simulink library "user_lib"  (R2022b)
settings: Solver=VariableStepAuto  StartTime=0.0  StopTime=10.0  RelTol=1e-3
libraries: simulink x5
settings Model: Creator=MBDUSR  LastModifiedBy=MBDUSR

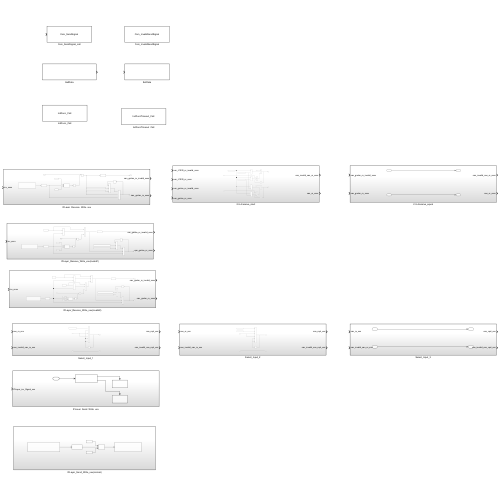
[thumbnail: Simulink's stored preview of the top-level diagram]
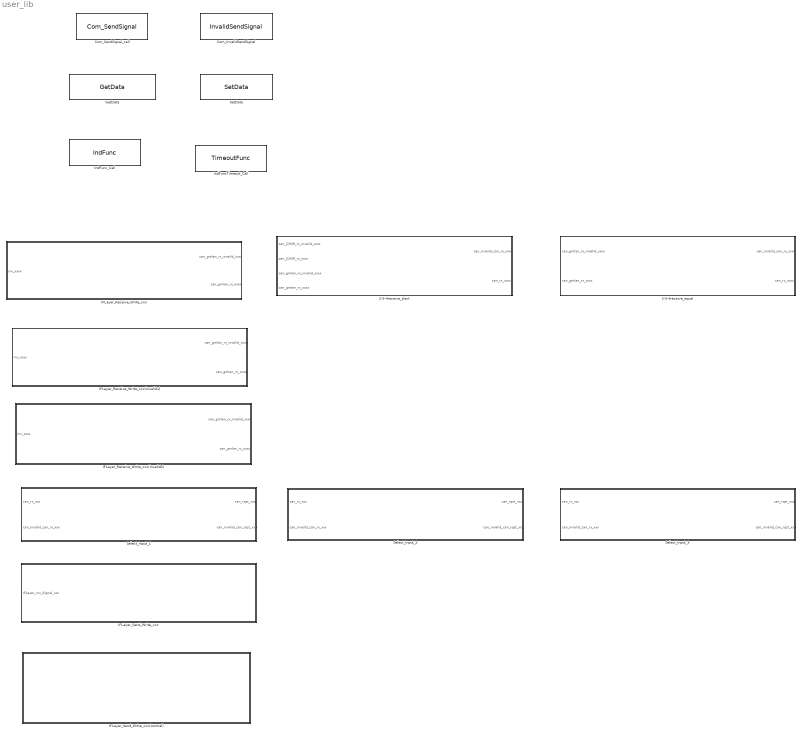
== system user_lib ==
  2-5-4receive_equal : Subsystem
  2-5-4receive_slect : Subsystem
  Com_InvalidSendSignal : S-Function  FunctionName=InvalidSendSignal  Parameters=signalId  SFunctionDeploymentMode=off  EnableBusSupport=off  mask{signalId=}
      mask Help: web('Com_InvalidSendSignal_help.html')
      mask DialogControl Container4 Prompt: Singal Parameter
      mask Display: disp('Com_InvalidSendSignal')
  Com_SendSignal_call : S-Function  FunctionName=Com_SendSignal  Parameters=signalId  SFunctionDeploymentMode=off  EnableBusSupport=off  mask{signalId=}
      mask Help: web('Com_SendSignal_help.html')
      mask DialogControl Container4 Prompt: Singal Parameter
      mask Display: disp('Com_SendSignal')
  GetData : S-Function  FunctionName=GetData  Parameters=interface,signalType  SFunctionDeploymentMode=off  EnableBusSupport=off  mask{interface=, signalType=UB}
      mask prompts: signalType "Signal Type"
      mask Help: web('GetData_help.html')
      mask TypeOptions signalType: UB | SB | UW | SW | UD | SD
      mask DialogControl Container4 Prompt: Singal Parameter
      mask Display:
      | interfaceName = get_param(gcbh, "interface");
      | s = strcat(interfaceName);
      | disp(s);
  IFLayer_Receive_Write_xxx : Subsystem
  IFLayer_Receive_Write_xxx(invalid1) : Subsystem
  IFLayer_Receive_Write_xxx(invalid2) : Subsystem
  IFLayer_Send_Write_xxx : Subsystem
  IFLayer_Send_Write_xxx(normal) : Subsystem
  IndFuncTimeout_Call : S-Function  FunctionName=TimeoutFunc  Parameters=siggroupIndex,canid,signalTable  SFunctionDeploymentMode=off  EnableBusSupport=off  mask{siggroupIndex=, canid=, signalTable={ 'UB', '', ''; 'UW', '', '' }}
      mask prompts: siggroupIndex "Signal Group Index"; canid "CAN ID"; signalTable "Signal Table"
      mask init:
      | %set_param(gcbh,'signalTable',{'1','signal1','index1'});
      mask Help: web('IndFuncTimeout_help.html')
      mask DialogControl Container4 Prompt: Singal Parameter
      mask Display: disp('IndFuncTimeout_Call')
  IndFunc_Call : S-Function  FunctionName=IndFunc  Parameters=siggroupIndex,canid,signalTable,timeoutflag,extendid  SFunctionDeploymentMode=off  EnableBusSupport=off  mask{siggroupIndex=, canid=, signalTable={ 'UB', '', ''; 'UB', '', '' }, timeoutflag=off, extendid=off}
      mask prompts: siggroupIndex "Signal Group Index"; canid "CAN ID"; signalTable "Signal Table"; timeoutflag "Timeout Flag"; extendid "Extend ID"
      mask init:
      | %set_param(gcbh,'signalTable',{'1','signal1','index1'});
      mask Help: web('IndFunc_help.html')
      mask DialogControl Container4 Prompt: Singal Parameter
      mask Display: disp('IndFunc_Call')
  Select_Input_1 : Subsystem
  Select_Input_2 : Subsystem
  Select_Input_3 : Subsystem
  SetData : S-Function  FunctionName=SetData  Parameters=interface  SFunctionDeploymentMode=off  EnableBusSupport=off  mask{interface=}
      mask Help: web('SetData_help.html')
      mask DialogControl Container4 Prompt: Singal Parameter
      mask Display:
      | interfaceName = get_param(gcbh, "interface");
      | s = strcat(interfaceName);
      | disp(s);

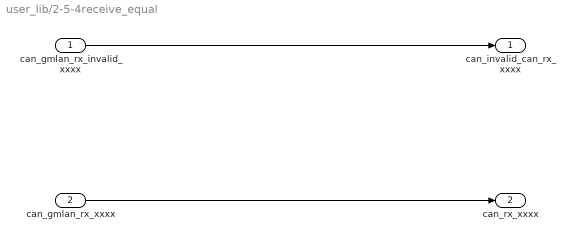
== system user_lib/2-5-4receive_equal ==
  can_gmlan_rx_invalid_xxxx : Inport
  can_gmlan_rx_xxxx : Inport  Port=2
  can_invalid_can_rx_xxxx : Outport
  can_rx_xxxx : Outport  Port=2
  wires:
  can_gmlan_rx_invalid_xxxx/1 -> can_invalid_can_rx_xxxx/1
  can_gmlan_rx_xxxx/1 -> can_rx_xxxx/1

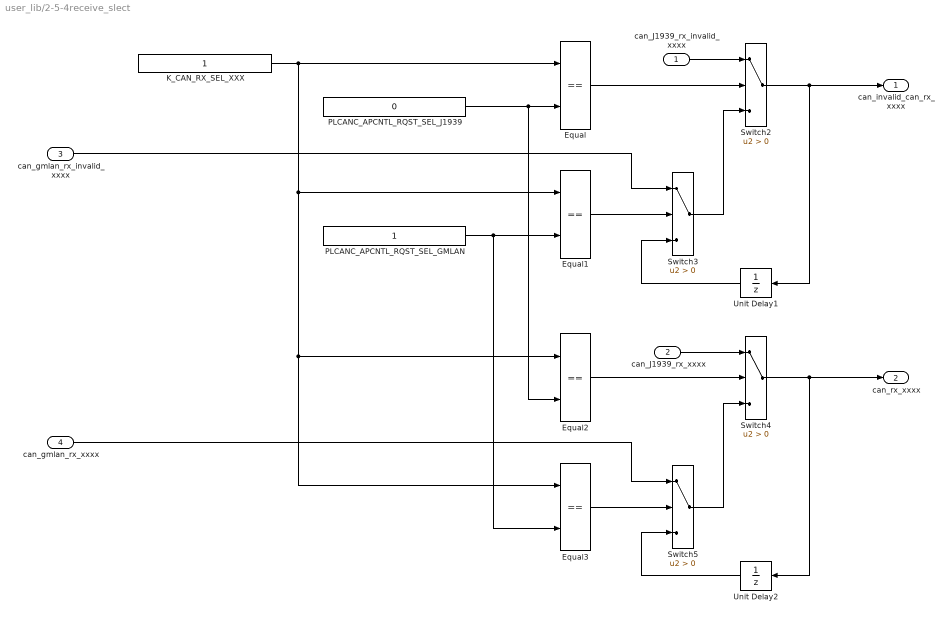
== system user_lib/2-5-4receive_slect ==
  can_J1939_rx_invalid_xxxx : Inport
  can_J1939_rx_xxxx : Inport  Port=2
  can_gmlan_rx_invalid_xxxx : Inport  Port=3
  can_gmlan_rx_xxxx : Inport  Port=4
  Equal{,1..3} (4 alike) : RelationalOperator  Operator===  OutDataTypeStr=boolean  RndMeth=Simplest  InputSameDT=off
  K_CAN_RX_SEL_XXX : Constant
  PLCANC_APCNTL_RQST_SEL_GMLAN : Constant
  PLCANC_APCNTL_RQST_SEL_J1939 : Constant  Value=0
  Switch{2..5} (4 alike) : Switch  Criteria=u2 > Threshold  SaturateOnIntegerOverflow=off  InputSameDT=off
  Unit Delay1 : UnitDelay  SampleTime=-1  HasFrameUpgradeWarning=on
  Unit Delay2 : UnitDelay  SampleTime=-1  HasFrameUpgradeWarning=on
  can_invalid_can_rx_xxxx : Outport
  can_rx_xxxx : Outport  Port=2
  wires:
  Equal/1 -> Switch2/2
  Unit Delay1/1 -> Switch3/3
  Switch2/1 -> Unit Delay1/1, can_invalid_can_rx_xxxx/1
  Unit Delay2/1 -> Switch5/3
  Equal1/1 -> Switch3/2
  Equal3/1 -> Switch5/2
  Switch5/1 -> Switch4/3
  can_gmlan_rx_invalid_xxxx/1 -> Switch3/1
  PLCANC_APCNTL_RQST_SEL_GMLAN/1 -> Equal3/2, Equal1/2
  can_J1939_rx_invalid_xxxx/1 -> Switch2/1
  Equal2/1 -> Switch4/2
  can_gmlan_rx_xxxx/1 -> Switch5/1
  PLCANC_APCNTL_RQST_SEL_J1939/1 -> Equal2/2, Equal/2
  Switch4/1 -> Unit Delay2/1, can_rx_xxxx/1
  K_CAN_RX_SEL_XXX/1 -> Equal3/1, Equal2/1, Equal1/1, Equal/1
  can_J1939_rx_xxxx/1 -> Switch4/1
  Switch3/1 -> Switch2/3

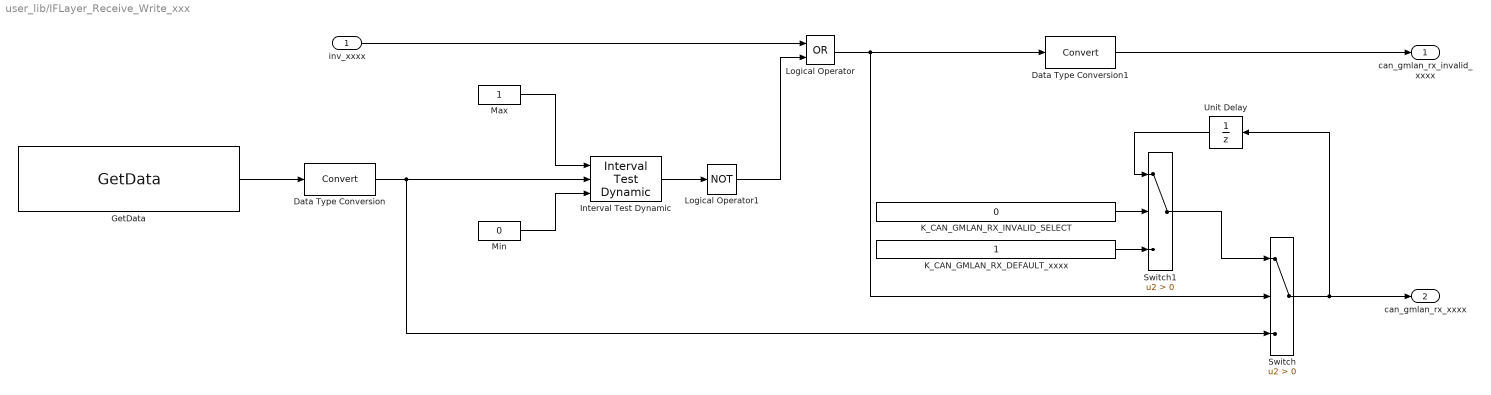
== system user_lib/IFLayer_Receive_Write_xxx ==
  inv_xxxx : Inport
  Data Type Conversion : DataTypeConversion  ConvertRealWorld=Stored Integer (SI)  SaturateOnIntegerOverflow=off  RndMeth=Floor
  Data Type Conversion1 : DataTypeConversion  ConvertRealWorld=Stored Integer (SI)  SaturateOnIntegerOverflow=off  RndMeth=Floor
  GetData : S-Function  FunctionName=GetData  Parameters=interface,signalType  SFunctionDeploymentMode=off  EnableBusSupport=off  mask{interface=, signalType=UB}
      mask prompts: signalType "Signal Type"
      mask TypeOptions signalType: UB | SB | UW | SW | UD | SD
      mask DialogControl Container4 Prompt: Singal Parameter
      mask Display:
      | interfaceName = get_param(gcbh, "interface");
      | s = strcat(interfaceName);
      | disp(s);
  Interval Test Dynamic : simulink/Logic and Bit Operations/Interval Test Dynamic  IntervalClosedRight=on  IntervalClosedLeft=on  OutDataTypeStr=boolean
  K_CAN_GMLAN_RX_DEFAULT_xxxx : Constant  OutDataTypeStr=Inherit: Inherit via back propagation
  K_CAN_GMLAN_RX_INVALID_SELECT : Constant  Value=0  OutDataTypeStr=Inherit: Inherit via back propagation
  Logical Operator : Logic  Operator=OR  AllPortsSameDT=off  OutDataTypeStr=boolean
  Logical Operator1 : Logic  Operator=NOT  AllPortsSameDT=off  OutDataTypeStr=boolean
  Max : Constant  OutDataTypeStr=Inherit: Inherit via back propagation
  Min : Constant  Value=0  OutDataTypeStr=Inherit: Inherit via back propagation
  Switch : Switch  Criteria=u2 > Threshold  SaturateOnIntegerOverflow=off  InputSameDT=off
  Switch1 : Switch  Criteria=u2 > Threshold  SaturateOnIntegerOverflow=off  InputSameDT=off
  Unit Delay : UnitDelay  SampleTime=-1  HasFrameUpgradeWarning=on
  can_gmlan_rx_invalid_xxxx : Outport
  can_gmlan_rx_xxxx : Outport  Port=2
  wires:
  Data Type Conversion/1 -> Interval Test Dynamic/2, Switch/3
  Interval Test Dynamic/1 -> Logical Operator1/1
  GetData/1 -> Data Type Conversion/1
  Unit Delay/1 -> Switch1/1
  Min/1 -> Interval Test Dynamic/3
  Max/1 -> Interval Test Dynamic/1
  Logical Operator1/1 -> Logical Operator/2
  Switch/1 -> Unit Delay/1, can_gmlan_rx_xxxx/1
  Switch1/1 -> Switch/1
  K_CAN_GMLAN_RX_DEFAULT_xxxx/1 -> Switch1/3
  Logical Operator/1 -> Switch/2, Data Type Conversion1/1
  Data Type Conversion1/1 -> can_gmlan_rx_invalid_xxxx/1
  K_CAN_GMLAN_RX_INVALID_SELECT/1 -> Switch1/2
  inv_xxxx/1 -> Logical Operator/1

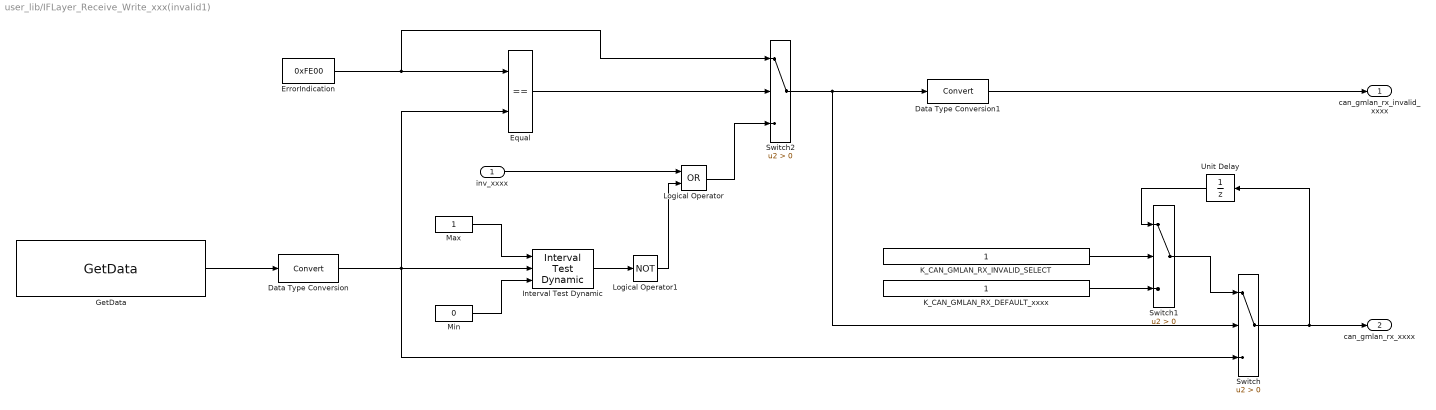
== system user_lib/IFLayer_Receive_Write_xxx(invalid1) ==
  inv_xxxx : Inport
  Data Type Conversion : DataTypeConversion  ConvertRealWorld=Stored Integer (SI)  SaturateOnIntegerOverflow=off  RndMeth=Floor
  Data Type Conversion1 : DataTypeConversion  ConvertRealWorld=Stored Integer (SI)  SaturateOnIntegerOverflow=off  RndMeth=Floor
  Equal : RelationalOperator  Operator===  OutDataTypeStr=boolean  RndMeth=Simplest  InputSameDT=off
  ErrorIndication : Constant  Value=0xFE00  OutDataTypeStr=Inherit: Inherit via back propagation
  GetData : S-Function  FunctionName=GetData  Parameters=interface,signalType  SFunctionDeploymentMode=off  EnableBusSupport=off  mask{interface=, signalType=UB}
      mask prompts: signalType "Signal Type"
      mask TypeOptions signalType: UB | SB | UW | SW | UD | SD
      mask DialogControl Container4 Prompt: Singal Parameter
      mask Display:
      | interfaceName = get_param(gcbh, "interface");
      | s = strcat(interfaceName);
      | disp(s);
  Interval Test Dynamic : simulink/Logic and Bit Operations/Interval Test Dynamic  IntervalClosedRight=on  IntervalClosedLeft=on  OutDataTypeStr=boolean
  K_CAN_GMLAN_RX_DEFAULT_xxxx : Constant  OutDataTypeStr=Inherit: Inherit via back propagation
  K_CAN_GMLAN_RX_INVALID_SELECT : Constant  OutDataTypeStr=Inherit: Inherit via back propagation
  Logical Operator : Logic  Operator=OR  AllPortsSameDT=off  OutDataTypeStr=boolean
  Logical Operator1 : Logic  Operator=NOT  AllPortsSameDT=off  OutDataTypeStr=boolean
  Max : Constant  OutDataTypeStr=Inherit: Inherit via back propagation
  Min : Constant  Value=0  OutDataTypeStr=Inherit: Inherit via back propagation
  Switch : Switch  Criteria=u2 > Threshold  SaturateOnIntegerOverflow=off  InputSameDT=off
  Switch1 : Switch  Criteria=u2 > Threshold  SaturateOnIntegerOverflow=off  InputSameDT=off
  Switch2 : Switch  Criteria=u2 > Threshold  SaturateOnIntegerOverflow=off  InputSameDT=off
  Unit Delay : UnitDelay  SampleTime=-1  HasFrameUpgradeWarning=on
  can_gmlan_rx_invalid_xxxx : Outport
  can_gmlan_rx_xxxx : Outport  Port=2
  wires:
  ErrorIndication/1 -> Equal/1, Switch2/1
  Data Type Conversion/1 -> Interval Test Dynamic/2, Switch/3, Equal/2
  Logical Operator/1 -> Switch2/3
  Equal/1 -> Switch2/2
  Switch2/1 -> Data Type Conversion1/1, Switch/2
  GetData/1 -> Data Type Conversion/1
  Interval Test Dynamic/1 -> Logical Operator1/1
  Logical Operator1/1 -> Logical Operator/2
  Data Type Conversion1/1 -> can_gmlan_rx_invalid_xxxx/1
  K_CAN_GMLAN_RX_INVALID_SELECT/1 -> Switch1/2
  Switch/1 -> can_gmlan_rx_xxxx/1, Unit Delay/1
  Min/1 -> Interval Test Dynamic/3
  Max/1 -> Interval Test Dynamic/1
  K_CAN_GMLAN_RX_DEFAULT_xxxx/1 -> Switch1/3
  inv_xxxx/1 -> Logical Operator/1
  Unit Delay/1 -> Switch1/1
  Switch1/1 -> Switch/1

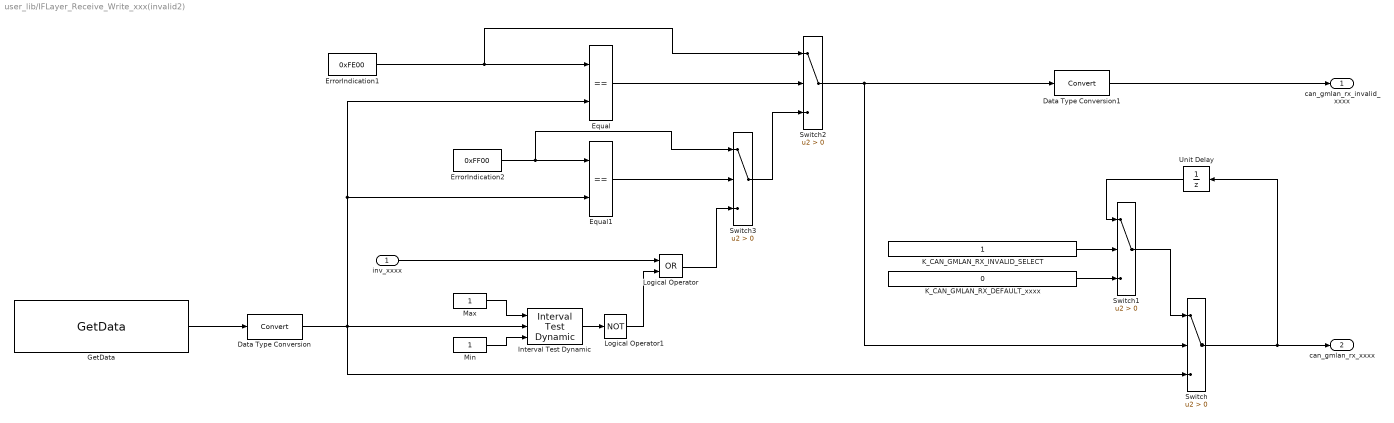
== system user_lib/IFLayer_Receive_Write_xxx(invalid2) ==
  inv_xxxx : Inport
  Data Type Conversion : DataTypeConversion  ConvertRealWorld=Stored Integer (SI)  SaturateOnIntegerOverflow=off  RndMeth=Floor
  Data Type Conversion1 : DataTypeConversion  ConvertRealWorld=Stored Integer (SI)  SaturateOnIntegerOverflow=off  RndMeth=Floor
  Equal : RelationalOperator  Operator===  OutDataTypeStr=boolean  RndMeth=Simplest  InputSameDT=off
  Equal1 : RelationalOperator  Operator===  OutDataTypeStr=boolean  RndMeth=Simplest  InputSameDT=off
  ErrorIndication1 : Constant  Value=0xFE00  OutDataTypeStr=Inherit: Inherit via back propagation
  ErrorIndication2 : Constant  Value=0xFF00  OutDataTypeStr=Inherit: Inherit via back propagation
  GetData : S-Function  FunctionName=GetData  Parameters=interface,signalType  SFunctionDeploymentMode=off  EnableBusSupport=off  mask{interface=, signalType=UB}
      mask prompts: signalType "Signal Type"
      mask TypeOptions signalType: UB | SB | UW | SW | UD | SD
      mask DialogControl Container4 Prompt: Singal Parameter
      mask Display:
      | interfaceName = get_param(gcbh, "interface");
      | s = strcat(interfaceName);
      | disp(s);
  Interval Test Dynamic : simulink/Logic and Bit Operations/Interval Test Dynamic  IntervalClosedRight=on  IntervalClosedLeft=on  OutDataTypeStr=boolean
  K_CAN_GMLAN_RX_DEFAULT_xxxx : Constant  Value=0  OutDataTypeStr=Inherit: Inherit via back propagation
  K_CAN_GMLAN_RX_INVALID_SELECT : Constant  OutDataTypeStr=Inherit: Inherit via back propagation
  Logical Operator : Logic  Operator=OR  AllPortsSameDT=off  OutDataTypeStr=boolean
  Logical Operator1 : Logic  Operator=NOT  AllPortsSameDT=off  OutDataTypeStr=boolean
  Max : Constant  OutDataTypeStr=Inherit: Inherit via back propagation
  Min : Constant  OutDataTypeStr=Inherit: Inherit via back propagation
  Switch{,1..3} (4 alike) : Switch  Criteria=u2 > Threshold  SaturateOnIntegerOverflow=off  InputSameDT=off
  Unit Delay : UnitDelay  SampleTime=-1  HasFrameUpgradeWarning=on
  can_gmlan_rx_invalid_xxxx : Outport
  can_gmlan_rx_xxxx : Outport  Port=2
  wires:
  ErrorIndication2/1 -> Equal1/1, Switch3/1
  ErrorIndication1/1 -> Equal/1, Switch2/1
  Data Type Conversion/1 -> Switch/3, Interval Test Dynamic/2, Equal/2, Equal1/2
  Switch3/1 -> Switch2/3
  Logical Operator/1 -> Switch3/3
  Equal1/1 -> Switch3/2
  GetData/1 -> Data Type Conversion/1
  Switch2/1 -> Switch/2, Data Type Conversion1/1
  Equal/1 -> Switch2/2
  Interval Test Dynamic/1 -> Logical Operator1/1
  Logical Operator1/1 -> Logical Operator/2
  Data Type Conversion1/1 -> can_gmlan_rx_invalid_xxxx/1
  K_CAN_GMLAN_RX_INVALID_SELECT/1 -> Switch1/2
  Switch/1 -> can_gmlan_rx_xxxx/1, Unit Delay/1
  Min/1 -> Interval Test Dynamic/3
  Max/1 -> Interval Test Dynamic/1
  K_CAN_GMLAN_RX_DEFAULT_xxxx/1 -> Switch1/3
  inv_xxxx/1 -> Logical Operator/1
  Unit Delay/1 -> Switch1/1
  Switch1/1 -> Switch/1

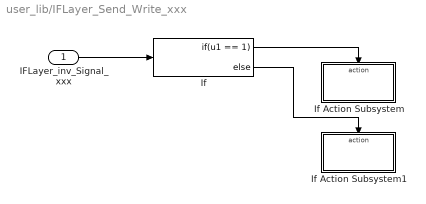
== system user_lib/IFLayer_Send_Write_xxx ==
  IFLayer_inv_Signal_xxx : Inport
  If : If  IfExpression=u1 == 1
  If Action Subsystem : Subsystem  TreatAsAtomicUnit=on
  If Action Subsystem1 : Subsystem  TreatAsAtomicUnit=on
  wires:
  If/2 -> If Action Subsystem1/Action
  If/1 -> If Action Subsystem/Action
  IFLayer_inv_Signal_xxx/1 -> If/1

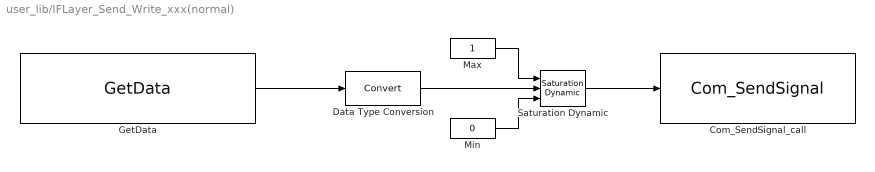
== system user_lib/IFLayer_Send_Write_xxx(normal) ==
  Com_SendSignal_call : S-Function  FunctionName=Com_SendSignal  Parameters=signalId  SFunctionDeploymentMode=off  EnableBusSupport=off  mask{signalId=}
      mask DialogControl Container4 Prompt: Singal Parameter
      mask Display: disp('Com_SendSignal')
  Data Type Conversion : DataTypeConversion  ConvertRealWorld=Stored Integer (SI)  SaturateOnIntegerOverflow=off  RndMeth=Floor
  GetData : S-Function  FunctionName=GetData  Parameters=interface,signalType  SFunctionDeploymentMode=off  EnableBusSupport=off  mask{interface=, signalType=UB}
      mask prompts: signalType "Signal Type"
      mask TypeOptions signalType: UB | SB | UW | SW | UD | SD
      mask DialogControl Container4 Prompt: Singal Parameter
      mask Display:
      | interfaceName = get_param(gcbh, "interface");
      | s = strcat(interfaceName);
      | disp(s);
  Max : Constant  OutDataTypeStr=Inherit: Inherit via back propagation
  Min : Constant  Value=0  OutDataTypeStr=Inherit: Inherit via back propagation
  Saturation Dynamic : simulink/Discontinuities/Saturation Dynamic  OutMin=[]  OutMax=[]  OutDataTypeStr=Inherit: Same as second input  OutDataType=fixdt(1, 16)  OutScaling=2^-10  DoSatur=off
  wires:
  Data Type Conversion/1 -> Saturation Dynamic/2
  GetData/1 -> Data Type Conversion/1
  Max/1 -> Saturation Dynamic/1
  Min/1 -> Saturation Dynamic/3
  Saturation Dynamic/1 -> Com_SendSignal_call/1

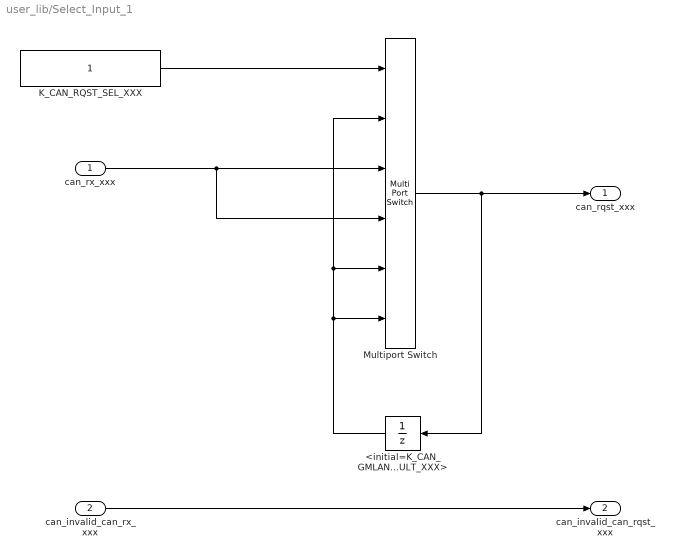
== system user_lib/Select_Input_1 ==
  can_rx_xxx : Inport
  can_invalid_can_rx_xxx : Inport  Port=2
  <initial=K_CAN_GMLAN_RX_DEFAULT_XXX> : UnitDelay  SampleTime=-1  HasFrameUpgradeWarning=on
  K_CAN_RQST_SEL_XXX : Constant
  Multiport Switch : MultiPortSwitch  DataPortOrder=Zero-based contiguous  Inputs=5  zeroidx=on  SaturateOnIntegerOverflow=off  InputSameDT=off
  can_rqst_xxx : Outport
  can_invalid_can_rqst_xxx : Outport  Port=2
  wires:
  can_invalid_can_rx_xxx/1 -> can_invalid_can_rqst_xxx/1
  can_rx_xxx/1 -> Multiport Switch/3, Multiport Switch/4
  Multiport Switch/1 -> <initial=K_CAN_GMLAN_RX_DEFAULT_XXX>/1, can_rqst_xxx/1
  <initial=K_CAN_GMLAN_RX_DEFAULT_XXX>/1 -> Multiport Switch/5, Multiport Switch/2, Multiport Switch/6
  K_CAN_RQST_SEL_XXX/1 -> Multiport Switch/1

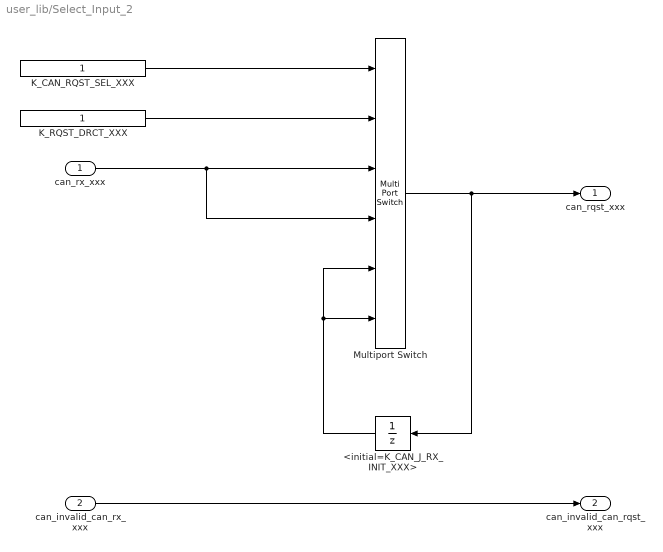
== system user_lib/Select_Input_2 ==
  can_rx_xxx : Inport
  can_invalid_can_rx_xxx : Inport  Port=2
  <initial=K_CAN_J_RX_INIT_XXX> : UnitDelay  SampleTime=-1  HasFrameUpgradeWarning=on
  K_CAN_RQST_SEL_XXX : Constant
  K_RQST_DRCT_XXX : Constant
  Multiport Switch : MultiPortSwitch  DataPortOrder=Zero-based contiguous  Inputs=5  zeroidx=on  SaturateOnIntegerOverflow=off  InputSameDT=off
  can_rqst_xxx : Outport
  can_invalid_can_rqst_xxx : Outport  Port=2
  wires:
  can_invalid_can_rx_xxx/1 -> can_invalid_can_rqst_xxx/1
  K_RQST_DRCT_XXX/1 -> Multiport Switch/2
  can_rx_xxx/1 -> Multiport Switch/3, Multiport Switch/4
  Multiport Switch/1 -> <initial=K_CAN_J_RX_INIT_XXX>/1, can_rqst_xxx/1
  <initial=K_CAN_J_RX_INIT_XXX>/1 -> Multiport Switch/5, Multiport Switch/6
  K_CAN_RQST_SEL_XXX/1 -> Multiport Switch/1

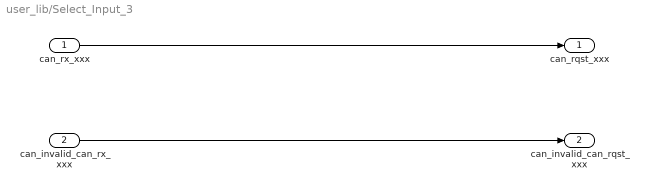
== system user_lib/Select_Input_3 ==
  can_rx_xxx : Inport
  can_invalid_can_rx_xxx : Inport  Port=2
  can_rqst_xxx : Outport
  can_invalid_can_rqst_xxx : Outport  Port=2
  wires:
  can_rx_xxx/1 -> can_rqst_xxx/1
  can_invalid_can_rx_xxx/1 -> can_invalid_can_rqst_xxx/1

== system user_lib/IFLayer_Send_Write_xxx/If Action Subsystem ==
  Action Port : ActionPort
  Com_InvalidSendSignal : S-Function  FunctionName=InvalidSendSignal  Parameters=signalId  SFunctionDeploymentMode=off  EnableBusSupport=off  mask{signalId=index2}
      mask DialogControl Container4 Prompt: Singal Parameter
      mask Display: disp('Com_InvalidSendSignal')

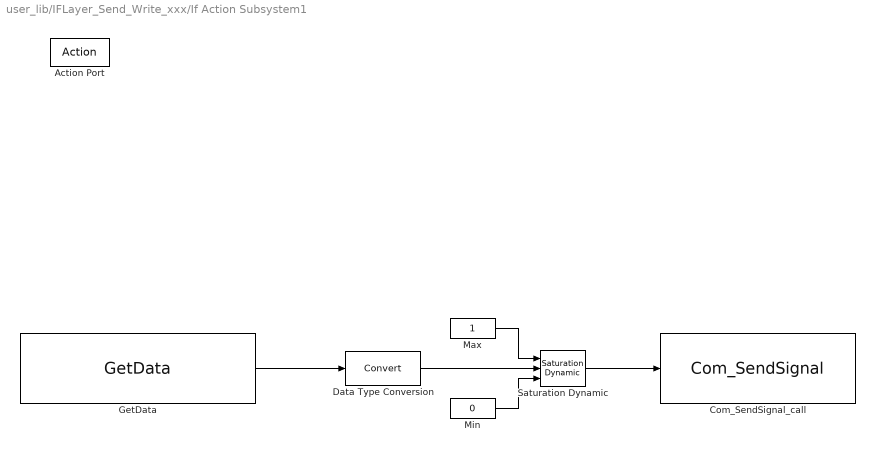
== system user_lib/IFLayer_Send_Write_xxx/If Action Subsystem1 ==
  Action Port : ActionPort
  Com_SendSignal_call : S-Function  FunctionName=Com_SendSignal  Parameters=signalId  SFunctionDeploymentMode=off  EnableBusSupport=off  mask{signalId=ComConfxxxTx}
      mask DialogControl Container4 Prompt: Singal Parameter
      mask Display: disp('Com_SendSignal')
  Data Type Conversion : DataTypeConversion  ConvertRealWorld=Stored Integer (SI)  SaturateOnIntegerOverflow=off  RndMeth=Floor
  GetData : S-Function  FunctionName=GetData  Parameters=interface,signalType  SFunctionDeploymentMode=off  EnableBusSupport=off  mask{interface=CIF_CO_INF_MENG_NOX_CALC_MGPMG, signalType=UB}
      mask prompts: signalType "Signal Type"
      mask TypeOptions signalType: UB | SB | UW | SW | UD | SD
      mask DialogControl Container4 Prompt: Singal Parameter
      mask Display:
      | interfaceName = get_param(gcbh, "interface");
      | s = strcat(interfaceName);
      | disp(s);
  Max : Constant  OutDataTypeStr=Inherit: Inherit via back propagation
  Min : Constant  Value=0  OutDataTypeStr=Inherit: Inherit via back propagation
  Saturation Dynamic : simulink/Discontinuities/Saturation Dynamic  OutMin=[]  OutMax=[]  OutDataTypeStr=Inherit: Same as second input  OutDataType=fixdt(1, 16)  OutScaling=2^-10  DoSatur=off
  wires:
  Max/1 -> Saturation Dynamic/1
  Data Type Conversion/1 -> Saturation Dynamic/2
  Min/1 -> Saturation Dynamic/3
  GetData/1 -> Data Type Conversion/1
  Saturation Dynamic/1 -> Com_SendSignal_call/1
